simulink model "Q6"  (R2015a)
settings: Solver=ode45  StartTime=0.0  StopTime=10.0  RelTol=1e-3
values from neighbouring files (symbols this model uses):
  A = [0 1;(m*g*l+(M*g*L/2)-k)/(((M*(L^2))/3)+m*(l^2)) -beta/J]    [12.m]    (also in lab3.m)
  B = [0 1]'    [12.m]    (also in lab3.m)
  C = [1 0;0 1]    [lab3.m]
  D = [0 0]'    [lab3.m]
  U = 0    [lab3.m]
  x0 = [pi/4 0]'    [12.m]    (also in lab3.m)
settings Model: Creator=Diogo  LastModifiedBy=Diogo

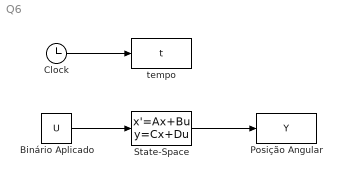
== system Q6 ==
  Binário Aplicado : Constant  Value=U
  Clock : Clock
  Posição Angular : ToWorkspace  VariableName=Y  SampleTime=0.001
  State-Space : StateSpace  A=A  B=B  C=C  D=D  X0=x0  ContinuousStateAttributes='Modelo'
  tempo : ToWorkspace  VariableName=t  SampleTime=0.001
  wires:
  Clock/1 -> tempo/1
  State-Space/1 -> Posição Angular/1
  Binário Aplicado/1 -> State-Space/1
